simulink model "smm_gait_control"  (R2018b)
settings: configuration reference "Configuration1khz" (kept outside this file)
InitFcn:
  | addpath('./functions/')
  | addpath('./policies/')
  | control_params
values from neighbouring files (symbols this model uses):
  rest = extract_policy_variables('policies/rest.mat')    [control_params.m]
  run_slow = extract_policy_variables('policies/06_run_reduced.mat')    [control_params.m]
  walk_slow = extract_policy_variables('policies/06_walk.mat')    [control_params.m]
undefined symbols (not defined in the file or in its folder): ctrl, Discrete, initial_dx_estimate, initial_dy_estimate, initial_dz_estimate, initial_z_estimate, sample_time, Time
libraries: simulink x42, ctrlSharedLib x7
(part 5 of 5)

== matlab function smm_gait_control/Behavior/Filtering/Kalman Filtering/Measurement Noise Covariance Matricies ==
  data: R_no_position output; R_transverse_right output; R_transverse_left output; vertical_GRF_L input; vertical_GRF_R input; sample_time parameter; ctrl parameter; R_vertical output
function [R_no_position, R_transverse_right, R_transverse_left, R_vertical] =...
         MeasurementNoiseCovariance(vertical_GRF_L, vertical_GRF_R, ...
         sample_time, ctrl)

    % filter states: [dx_w]; [dy_w]; [dz_w];
    % measurements:  [dx_w-dfL + dfL_hat; dx_w-dfR + dfR_hat]; 

    ratio_L = max(0, min(vertical_GRF_L/(ctrl.kalman_stance_slip_threshold*ctrl.m_total*ctrl.g),1)); % ratio is 0 if no load, 1 if at least equilibrium
    ratio_R = max(0, min(vertical_GRF_R/(ctrl.kalman_stance_slip_threshold*ctrl.m_total*ctrl.g),1));
    R_transverse_right = diag([ratio_R*ctrl.R_kalman_foot_stance + (1-ratio_R)*ctrl.R_kalman_foot_slip, ...
                               ctrl.R_kalman_accelerometer])/sample_time;
    R_transverse_left = diag([ratio_L*ctrl.R_kalman_foot_stance + (1-ratio_L)*ctrl.R_kalman_foot_slip, ...
                              ctrl.R_kalman_accelerometer])/sample_time;            
    R_vertical = diag([ratio_L*ctrl.R_kalman_foot_stance  + (1-ratio_L)*ctrl.R_kalman_foot_slip,...
                       ratio_R*ctrl.R_kalman_foot_stance  + (1-ratio_R)*ctrl.R_kalman_foot_slip,...
                       ctrl.R_kalman_accelerometer])/sample_time;
                   
    R_no_position = diag([ratio_L*ctrl.R_kalman_dfoot_stance + (1-ratio_L)*ctrl.R_kalman_dfoot_slip, ...
                          ratio_R*ctrl.R_kalman_dfoot_stance + (1-ratio_R)*ctrl.R_kalman_dfoot_slip, ...
                          ctrl.R_kalman_accelerometer])/sample_time;
end

== matlab function smm_gait_control/Behavior/Convert to Body Frame IMU Accelerations ==
  data: accelerometer input; imu_accelerations output; ctrl parameter
function imu_accelerations = imu_to_body_frame(accelerometer, ctrl)
    z_up_rotation = [1, 0, 0; 0, 0, 1; 0, -1, 0];
    align_xy_rotation = [sqrt(2)/2, -sqrt(2)/2, 0; sqrt(2)/2, sqrt(2)/2, 0; 0, 0, 1];
    imu_accelerations = ctrl.g*z_up_rotation*align_xy_rotation*accelerometer;
end

== matlab function smm_gait_control/Behavior/Motion Planner/Plan Swing Leg Trajectories/Plan Swing Trajectories ==
  data: enable input; replan input; angle_of_attack input; touchdown_will_occur input; plan_length input; stance_plan_timings input size=[ctrl.max_trajectory_length 1]; stance_state_plan input size=[ctrl.max_trajectory_length 6]; double_support_time input; t_plan input; section_number input; phase input; com_x_velocity input; z_state input; foot2com_x_primary input; foot2com_z_primary input; foot2com_x_secondary input; foot2com_z_secondary input; right_is_primary input; gait_id input; neutral_point input; k_placement input; desired_x_primary output; desired_y_primary output; desired_z_primary output; desired_x_secondary output; desired_y_secondary output; desired_z_secondary output; ctrl parameter; walk_slow parameter; run_slow parameter; rest parameter
% Plan Foot2CoM trajectories in XYZ space for the swing phase
function [desired_x_primary, desired_y_primary, desired_z_primary, ...
          desired_x_secondary, desired_y_secondary, desired_z_secondary] = ...
          PlanFeet(enable, replan, angle_of_attack, touchdown_will_occur, ...
                    plan_length, stance_plan_timings, stance_state_plan, double_support_time, t_plan, ...
                    section_number, phase, com_x_velocity, z_state, ...
                    foot2com_x_primary, foot2com_z_primary, ...
                    foot2com_x_secondary, foot2com_z_secondary, ...
                    right_is_primary, gait_id, neutral_point, k_placement, ...
                    ctrl, walk_slow, run_slow, rest)
                  
  % not applicable in double support (return zero)
  if phase == 2
    desired_x_primary = [0 0 0]';
    desired_y_primary = [0 0 0]';
    desired_z_primary = [0 0 0]';
    desired_x_secondary = [0 0 0]';
    desired_y_secondary = [0 0 0]';
    desired_z_secondary = [0 0 0]';
    return;
  end
  
  % select gait dependent parameters
  switch(gait_id)
    case 1
      com_x_vel_desired = rest.desired_x_velocity;
      rest_length = rest.model.l0;
    case 2
      com_x_vel_desired = walk_slow.desired_x_velocity;
      rest_length = walk_slow.model.l0;
    case 3
      com_x_vel_desired = run_slow.desired_x_velocity;
      rest_length = run_slow.model.l0;
    otherwise
      com_x_vel_desired = run_slow.desired_x_velocity;
      rest_length = run_slow.model.l0;
  end
  
  % persistent variables to store swing foot plan(s) as splines in (X,Z) space
  persistent ax1 bx1 cx1 dx1 ax2 bx2 cx2 dx2 az1 bz1 cz1 dz1 az2 bz2 cz2 dz2 ...
             t_final x0_secondary_pos x0_secondary_vel

  % plan swing feet
  if isempty(ax1) || replan
    % convert (leg_length, leg_angle) space to (X,Z) space
    x_target = -rest_length * cosd(angle_of_attack);
    z_target =  rest_length * sind(angle_of_attack);
    if section_number == 1 % Flight (plan primary and secondary legs)
      % calculate swing time in flight
      t_final = (z_state(2) + sqrt(max(z_state(2)^2 - 2*ctrl.g*(z_target-z_state(1)),0)))/ctrl.g;
      t_min = abs(z_target - foot2com_z_primary(1)) / ctrl.max_vert_swing_speed;
      t_final = max(t_final, t_min); % lower bound swing time
      % primary x trajectory during flight
      x0_primary_pos = foot2com_x_primary(1); 
      x0_primary_vel = foot2com_x_primary(2);
      xf_pos = x_target;
      xf_vel = com_x_velocity; % match horizontal ground speed in flight
      [ ax1, bx1, cx1, dx1 ] = FindCubicCoefficients( x0_primary_pos, x0_primary_vel, ...
                                                      xf_pos, xf_vel, t_final );
      % secondary x trajectory during flight (symmetric about x = 0)
      x0_secondary_pos = foot2com_x_secondary(1); 
      x0_secondary_vel = foot2com_x_secondary(2);
      xf_pos = -x_target;
      xf_vel = 0;
      [ ax2, bx2, cx2, dx2 ] = FindCubicCoefficients( x0_secondary_pos, x0_secondary_vel, ...
                                                      xf_pos, xf_vel, t_final );
      % primary z trajectory during flight
      z0_pos = foot2com_z_primary(1);
      z0_vel = foot2com_z_primary(2);
      zf_pos = z_target;
      zf_vel = 0;
      [ az1, bz1, cz1, dz1 ] = FindCubicCoefficients( z0_pos, z0_vel, zf_pos, zf_vel, t_final );
      % secondary z trajectory during flight
      z0_pos = foot2com_z_secondary(1);
      z0_vel = foot2com_z_secondary(2);
      zf_pos = z_target - ctrl.z_retract_flight;
      zf_vel = 0;
      [ az2, bz2, cz2, dz2 ] = FindCubicCoefficients( z0_pos, z0_vel, zf_pos, zf_vel, t_final );
    elseif section_number == 2 % single support initial (SSI)
      final_stance_time = stance_plan_timings(plan_length);
      % plan targets based on if transitioning to double support or flight
      if touchdown_will_occur % to double support phase
        t_final = max(double_support_time, ctrl.min_swing_time);
        zmid_retract = 0.5 * ctrl.retract_extend_speed * t_final; % approximation
        zmid_retract = max(min(zmid_retract, ctrl.max_z_retract), ctrl.min_z_retract);
        zf_pos = z_target;
      else                    % to flight phase
        t_final = final_stance_time; 
        zmid_retract = ctrl.z_retract_flight;
        zf_pos = stance_state_plan(plan_length,3) - 0.30*zmid_retract;
      end
      % secondary x trajectory
      x0_secondary_pos = foot2com_x_secondary(1); 
      x0_secondary_vel = foot2com_x_secondary(2);
      xf_pos = x_target;
      xf_vel = 0;
      [ ax1, bx1, cx1, dx1 ] = FindCubicCoefficients( x0_secondary_pos, x0_secondary_vel, ...
                                                      xf_pos, xf_vel, t_final );
      ax2 = 0; bx2 = 0; cx2 = 0; dx2 = 0;
      % (retract/extend from SSI) 
      % secondary z trajectory (first half, retraction)
      z0_pos = foot2com_z_secondary(1);
      z0_vel = foot2com_z_secondary(2);
      zmid_pos = interp1(stance_plan_timings(1:plan_length), stance_state_plan(1:plan_length,3), ...
                         min(0.5*t_final, final_stance_time),'linear') - zmid_retract;
      zmid_vel = 0;
      [ az1, bz1, cz1, dz1 ] = FindCubicCoefficients( z0_pos, z0_vel, zmid_pos, zmid_vel, 0.5*t_final );
      % secondary z trajectory (second half, extension)
      zf_vel = 0;
      [ az2, bz2, cz2, dz2 ] = FindCubicCoefficients( zmid_pos, zmid_vel, zf_pos, zf_vel, 0.5*t_final );
    else % section_number == 3, single support apex (SSA)
      % plan until initial double support
      min_time = abs(z_target - foot2com_z_secondary(1)) / ctrl.retract_extend_speed;
      t_final = max(double_support_time, min_time);
      % secondary x trajectory
      x0_secondary_pos = foot2com_x_secondary(1); 
      x0_secondary_vel = foot2com_x_secondary(2);
      xf_pos = x_target;
      xf_vel = 0;
      [ ax1, bx1, cx1, dx1 ] = FindCubicCoefficients( x0_secondary_pos, x0_secondary_vel, ...
                                                      xf_pos, xf_vel, t_final );
      ax2 = 0; bx2 = 0; cx2 = 0; dx2 = 0;
      % secondary z trajectory (only extend from SSA)
      z0_pos = foot2com_z_secondary(1);
      z0_vel = foot2com_z_secondary(2);
      zf_vel = 0;
      [ az1, bz1, cz1, dz1 ] = FindCubicCoefficients( z0_pos, z0_vel, z_target, zf_vel, t_final );
      az2 = 0; bz2 = 0; cz2 = 0; dz2 = 0;
    end
  end
  
  % y target varies from left to right side of robot
  if right_is_primary
    y_swing_target_1 = ctrl.y_swing_target_right;
    y_swing_target_2 = ctrl.y_swing_target_left;
  else
    y_swing_target_1 = ctrl.y_swing_target_left;
    y_swing_target_2 = ctrl.y_swing_target_right;
  end
  
  % compute reference from polynomials if enabled
  if enable
    % bound the time
    trajectory_valid = t_plan <= t_final;
    t_plan = min(max(t_plan,0),t_final);
%     % replan using feedback policy
%     if phase == 1 && touchdown_will_occur
%        %xf_pos = neutral_point + k_placement * (com_x_vel_desired - com_x_velocity);
%        xf_pos = -0.25 + 0.10 * (com_x_vel_desired - com_x_velocity);
%        xf_pos = min(max(xf_pos, -0.5), 0.5);
%        xf_vel = 0;
%       [ ax1, bx1, cx1, dx1 ] = FindCubicCoefficients( x0_secondary_pos, x0_secondary_vel, xf_pos, xf_vel, t_final );
%     end
    % compute x reference
    x_pos = ax1*t_plan^3 + bx1*t_plan^2 + cx1*t_plan + dx1;
    x_vel = trajectory_valid*(3*ax1*t_plan^2 + 2*bx1*t_plan + cx1);
    x_acc = trajectory_valid*(6*ax1*t_plan + 2*bx1);
    % compute other references in flight
    if phase == 0
        x_pos_2 = ax2*t_plan^3 + bx2*t_plan^2 + cx2*t_plan + dx2;
        x_vel_2 = trajectory_valid*(3*ax2*t_plan^2 + 2*bx2*t_plan + cx2);
        x_acc_2 = trajectory_valid*(6*ax2*t_plan + 2*bx2);
        z_pos_1 = az1*t_plan^3 + bz1*t_plan^2 + cz1*t_plan + dz1;
        z_vel_1 = trajectory_valid*(3*az1*t_plan^2 + 2*bz1*t_plan + cz1);
        z_acc_1 = trajectory_valid*(6*az1*t_plan + 2*bz1);
        z_pos_2 = az2*t_plan^3 + bz2*t_plan^2 + cz2*t_plan + dz2;
        z_vel_2 = trajectory_valid*(3*az2*t_plan^2 + 2*bz2*t_plan + cz2);
        z_acc_2 = trajectory_valid*(6*az2*t_plan + 2*bz2); 
        % assign references to outputs
        desired_x_primary = [x_pos; x_vel; x_acc];
        desired_y_primary = [y_swing_target_1; 0; 0];
        desired_z_primary = [z_pos_1; z_vel_1; z_acc_1];
        desired_x_secondary = [x_pos_2; x_vel_2; x_acc_2];
        desired_y_secondary = [y_swing_target_2; 0; 0];
        desired_z_secondary = [z_pos_2; z_vel_2; z_acc_2];
    else % compute z references in single support
      if section_number == 2
        if t_plan < 0.5*t_final % retraction (always retract)
          z_pos = az1*t_plan^3 + bz1*t_plan^2 + cz1*t_plan + dz1;
          z_vel = trajectory_valid*(3*az1*t_plan^2 + 2*bz1*t_plan + cz1);
          z_acc = trajectory_valid*(6*az1*t_plan + 2*bz1); 
        else % extension
          t_plan = t_plan - 0.5*t_final;
          z_pos = az2*t_plan^3 + bz2*t_plan^2 + cz2*t_plan + dz2;
          z_vel = trajectory_valid*(3*az2*t_plan^2 + 2*bz2*t_plan + cz2);
          z_acc = trajectory_valid*(6*az2*t_plan + 2*bz2);
        end
      else % section_number == 3
        z_pos = az1*t_plan^3 + bz1*t_plan^2 + cz1*t_plan + dz1;
        z_vel = trajectory_valid*(3*az1*t_plan^2 + 2*bz1*t_plan + cz1);
        z_acc = trajectory_valid*(6*az1*t_plan + 2*bz1); 
      end
      if touchdown_will_occur && ~trajectory_valid
        z_pos = z_pos + 0.05;
      end
      % assign references to outputs
      desired_x_primary = [0; 0; 0];
      desired_y_primary = [0; 0; 0];
      desired_z_primary = [0; 0; 0];
      desired_x_secondary = [x_pos; x_vel; x_acc];
      desired_y_secondary = [y_swing_target_2; 0; 0];
      desired_z_secondary = [z_pos; z_vel; z_acc];
    end

  else % Use static targets otherwise
    desired_y_primary = [y_swing_target_1 0 0]';
    desired_y_secondary = [y_swing_target_2 0 0]';
    
    % single support static target
    desired_x_primary = [ctrl.static_single_x_pos_swing 0 0]';
    desired_z_primary = [ctrl.static_single_z_pos_swing 0 0]';
    desired_x_secondary = -desired_x_primary;
    desired_z_secondary = desired_z_primary - ctrl.z_retract_flight;
    
    % double support static target
    if gait_id == 1
      desired_z_primary = [ctrl.static_double_z_pos_swing 0 0]';
      desired_z_secondary = desired_z_primary;
      if phase == 1 % single support
        desired_x_primary = [0; 0; 0];
        desired_x_secondary = [-sign(foot2com_x_primary(1)) * abs(ctrl.static_double_x_pos_swing); 0; 0];
      else          % flight
        desired_x_primary = [ctrl.static_double_x_pos_swing 0 0]';
        desired_x_secondary = -desired_x_primary;
      end
    end
    
  end
  
end

== matlab function smm_gait_control/Behavior/SEA Measurements/Leg Dynamics Left ==
  data: tau_back input; tau_front input; axial_force output; leg_width input; leg_length input; ortho_force output
function [axial_force, ortho_force] = fcn(tau_back, tau_front, leg_width, leg_length)

  % prevent divide by zero
  leg_width(1) = max(leg_width(1),eps);
  leg_length(1) = max(leg_length(1),eps);

  % forces and torques
  hip_torque = tau_front + tau_back;
  spread_torque = tau_front - tau_back;
  axial_force = zeros(2,1);
  axial_force(1) = spread_torque(1) / leg_width(1);
  ortho_force = zeros(2,1);
  ortho_force(1) = hip_torque(1) / leg_length(1);
  
  % time derivatives
  axial_force(2) = (leg_width(1)*spread_torque(2) - spread_torque(1)*leg_width(2)) / (leg_width(1)*leg_width(1));
  ortho_force(2) = (leg_length(1)*hip_torque(2) - hip_torque(1)*leg_length(2)) / (leg_length(1)*leg_length(1));
  
end

== matlab function smm_gait_control/Behavior/Leg Plane GRF Right/World Frame React Forces ==
  data: F_horz output; leg_angle input; F_vert output; torso_pitch input; F_axial input; F_ortho input
function [F_horz, F_vert] = fcn(leg_angle, torso_pitch, F_axial, F_ortho)

  % define world frame leg angle
  gamma = leg_angle + torso_pitch;

  % compute forces
  F_vert = zeros(2,1);
  F_horz = zeros(2,1);
  F_vert(1) = -F_axial(1)*cos(gamma(1)) + F_ortho(1)*sin(gamma(1));
  F_horz(1) = -F_axial(1)*sin(gamma(1)) - F_ortho(1)*cos(gamma(1));
  
  % compute time derivatives
  F_vert(2) =  gamma(2)*(F_axial(1)*sin(gamma(1)) + F_ortho(1)*cos(gamma(1))) - F_axial(2)*cos(gamma(1)) + F_ortho(2)*sin(gamma(1));
  F_horz(2) =  gamma(2)*(-F_axial(1)*cos(gamma(1)) + F_ortho(1)*sin(gamma(1))) - F_axial(2)*sin(gamma(1)) - F_ortho(2)*cos(gamma(1));
  
end

== matlab function smm_gait_control/Behavior/Leg Plane GRF Left/World Frame React Forces ==
  data: F_horz output; leg_angle input; F_vert output; torso_pitch input; F_axial input; F_ortho input
function [F_horz, F_vert] = fcn(leg_angle, torso_pitch, F_axial, F_ortho)

  % define world frame leg angle
  gamma = leg_angle + torso_pitch;

  % compute forces
  F_vert = zeros(2,1);
  F_horz = zeros(2,1);
  F_vert(1) = -F_axial(1)*cos(gamma(1)) + F_ortho(1)*sin(gamma(1));
  F_horz(1) = -F_axial(1)*sin(gamma(1)) - F_ortho(1)*cos(gamma(1));
  
  % compute time derivatives
  F_vert(2) =  gamma(2)*(F_axial(1)*sin(gamma(1)) + F_ortho(1)*cos(gamma(1))) - F_axial(2)*cos(gamma(1)) + F_ortho(2)*sin(gamma(1));
  F_horz(2) =  gamma(2)*(-F_axial(1)*cos(gamma(1)) + F_ortho(1)*sin(gamma(1))) - F_axial(2)*sin(gamma(1)) - F_ortho(2)*cos(gamma(1));
  
end

== matlab function smm_gait_control/Behavior/Swing Leg Control Secondary/Virtual Leg to Four Bar ==
  data: l_leg input; dl_leg input; ddl_leg input; phi input; dphi input; ddphi input; back output; dback output; ddback output; front output; dfront output; ddfront output
function [back, dback, ddback, front, dfront, ddfront] = VirtualLegToFourBar(l_leg, dl_leg, ddl_leg, phi, dphi, ddphi)
    [back, dback, ddback, front, dfront, ddfront] = VirtualLegToFourBar(l_leg, dl_leg, ddl_leg, phi, dphi, ddphi);
end

== matlab function smm_gait_control/Behavior/CoM Kinematics/PositionUsingRobotGeometry ==
  data: com_left_yawed output; dcom_left_yawed output; com_right_yawed output; dcom_right_yawed output; roll input; pitch input; yaw input; left_leg_sagittal_angle input; left_leg_lateral_angle input; left_leg_length input; right_leg_sagittal_angle input; right_leg_lateral_angle input; right_leg_length input; com_left_global output; dcom_left_global output; ctrl parameter; com_right_global output; dcom_right_global output; com_pelvis_body output; dcom_pelvis_body output
% Returns CoM relative to primary foot
function [com_left_yawed, dcom_left_yawed, ...
          com_right_yawed, dcom_right_yawed, ...
          com_left_global, dcom_left_global, ...
          com_right_global, dcom_right_global, ...
          com_pelvis_body, dcom_pelvis_body] = ...
         ComPositionUsingRobotGeometry(roll, pitch, yaw, ...
                           left_leg_sagittal_angle, left_leg_lateral_angle, left_leg_length, ...
                           right_leg_sagittal_angle, right_leg_lateral_angle, right_leg_length, ...
                           ctrl)
                    
  q =  [roll(1), pitch(1), yaw(1), ...
        left_leg_sagittal_angle(1), left_leg_lateral_angle(1), left_leg_length(1), ...
        right_leg_sagittal_angle(1), right_leg_lateral_angle(1), right_leg_length(1)];
  dq = [roll(2), pitch(2), yaw(2), ...
        left_leg_sagittal_angle(2), left_leg_lateral_angle(2), left_leg_length(2), ...
        right_leg_sagittal_angle(2), right_leg_lateral_angle(2), right_leg_length(2)];

  [ com_pelvis, dcom_pelvis, ...
    com_left, dcom_left, ...
    com_right, dcom_right ] = ...
  ComCalculationFromRobot( q, dq, ctrl.m_torso, ctrl.m_leg_motor, ctrl.m_leg, ctrl.com_torso, ...
                           ctrl.com_leg_motor, ctrl.lateral_offset );
  
  % left foot measurements
  com_left_yawed = com_left(4:6);
  com_left_global = com_left(7:9);
  dcom_left_yawed = dcom_left(4:6);
  dcom_left_global = dcom_left(7:9);
  
  % right foot measurements
  com_right_yawed = com_right(4:6);
  com_right_global = com_right(7:9);
  dcom_right_yawed = dcom_right(4:6);
  dcom_right_global = dcom_right(7:9);
  
  % pelvis measurement
  com_pelvis_body = com_pelvis(1:3);
  dcom_pelvis_body = dcom_pelvis(1:3);
  
end

== matlab function smm_gait_control/Behavior/Primary-Secondary Routing Outputs ==
  data: right_is_primary input size=1; joint_torque_primary input size=2; motor_velocity_primary input size=2; lateral_torque_primary input size=1; joint_torque_secondary input size=2; motor_velocity_secondary input size=2; lateral_torque_secondary input size=1; joint_torque_right output size=2; motor_velocity_right output size=2; lateral_torque_right output size=1; joint_torque_left output size=2; motor_velocity_left output size=2; lateral_torque_left output size=1
% Switch between "primary" and "secondary" leg variables
function [joint_torque_right, ...
          motor_velocity_right, ...
          lateral_torque_right, ...
          joint_torque_left, ...
          motor_velocity_left, ...
          lateral_torque_left] ...
          = SignalSwitch(...
          right_is_primary, ...
          joint_torque_primary, ...
          motor_velocity_primary, ...
          lateral_torque_primary, ...
          joint_torque_secondary, ...
          motor_velocity_secondary, ...
          lateral_torque_secondary)

if right_is_primary % right leg is primary
  joint_torque_right = joint_torque_primary;
  motor_velocity_right = motor_velocity_primary;
  lateral_torque_right = lateral_torque_primary;
  joint_torque_left = joint_torque_secondary;
  motor_velocity_left = motor_velocity_secondary;
  lateral_torque_left = lateral_torque_secondary;
else % left leg is primary
  joint_torque_right = joint_torque_secondary;
  motor_velocity_right = motor_velocity_secondary;
  lateral_torque_right = lateral_torque_secondary;
  joint_torque_left = joint_torque_primary;
  motor_velocity_left = motor_velocity_primary;
  lateral_torque_left = lateral_torque_primary;
end

== matlab function smm_gait_control/Behavior/Swing Leg Control Primary/Avoid Hitting Mechanical Limits ==
  data: back_cmd output double; front_cmd output double; dback_cmd output double; dfront_cmd output double; ddback_cmd output double; ddfront_cmd output double; back_desired input; dback_desired input; ddback_desired input; front_desired input; dfront_desired input; ddfront_desired input; ctrl parameter
%% Avoid fourbar limits by saturating the commands and ensuring we don't command velocities or 
% accelerations that would push us into the limits when nearby
function [back_cmd, front_cmd, dback_cmd, dfront_cmd, ddback_cmd, ddfront_cmd] ...
    = AvoidFourbarLimits(back_desired,dback_desired, ddback_desired, ...
          front_desired, dfront_desired, ddfront_desired, ...
          ctrl)
    [back_cmd, front_cmd, dback_cmd, dfront_cmd, ddback_cmd, ddfront_cmd] = ...
      AvoidFourbarLimits(back_desired, dback_desired, ddback_desired, ...
                         front_desired, dfront_desired, ddfront_desired, ...
                         ctrl.min_front_bar_angle, ctrl.max_front_bar_angle, ...
                         ctrl.min_back_bar_angle, ctrl.max_back_bar_angle);
end

== matlab function smm_gait_control/Behavior/Swing Leg Control Secondary/Avoid Virtual Leg Length Limits ==
  data: l_leg_desired input; dl_leg_desired input; ddl_leg_desired input; l_leg_cmd output double; dl_leg_cmd output double; ddl_leg_cmd output double; ctrl parameter
%% Avoid virtual leg length limits by ensuring we don't command position/velocities/accelerations that would hit them.
function [l_leg_cmd, dl_leg_cmd, ddl_leg_cmd] = ...
  AvoidVirtualLengthLimits(l_leg_desired, dl_leg_desired, ddl_leg_desired, ctrl)
    [l_leg_cmd, dl_leg_cmd, ddl_leg_cmd] = ...
      AvoidVirtualLengthLimits(l_leg_desired, dl_leg_desired, ddl_leg_desired, ...
                               ctrl.min_leg_length, ctrl.max_leg_length);
end

== matlab function smm_gait_control/Behavior/Swing Leg Control Primary/Avoid Virtual Leg Length Limits ==
  data: l_leg_desired input; dl_leg_desired input; ddl_leg_desired input; l_leg_cmd output double; dl_leg_cmd output double; ddl_leg_cmd output double; ctrl parameter
%% Avoid virtual leg length limits by ensuring we don't command position/velocities/accelerations that would hit them.
function [l_leg_cmd, dl_leg_cmd, ddl_leg_cmd] = ...
  AvoidVirtualLengthLimits(l_leg_desired, dl_leg_desired, ddl_leg_desired, ctrl)
    [l_leg_cmd, dl_leg_cmd, ddl_leg_cmd] = ...
      AvoidVirtualLengthLimits(l_leg_desired, dl_leg_desired, ddl_leg_desired, ...
                               ctrl.min_leg_length, ctrl.max_leg_length);
end

== matlab function smm_gait_control/Behavior/Swing Leg Control Primary/Convert CoM (X,Y,Z) to  (Leg Angles, Leg Length) ==
  data: desired_leg_length output; X_star input; Y_star input; Z_star input; right_left input; pelvis2com_pos input; desired_alpha output; desired_beta output; pelvis2com_vel input; roll input; pitch input; sagittal_angle input; lateral_angle input; leg_length input; ctrl parameter
%% Convert Foot2CoM vector from (X, Y, Z) to (leg length, leg angle) space
function [ desired_leg_length, desired_alpha, desired_beta ]  =  ...
          ConvertToJointAnglesAndLegLength(X_star, Y_star, Z_star, right_left,...
                           pelvis2com_pos, pelvis2com_vel, ...
                           roll, pitch, sagittal_angle, lateral_angle, leg_length,...
                           ctrl) 

    q = [roll(1), pitch(1), sagittal_angle(1), lateral_angle(1), leg_length(1)];
    dq = [roll(2), pitch(2), sagittal_angle(2), lateral_angle(2), leg_length(2)];
    [desired_alpha, desired_beta, desired_leg_length] = ...
      ConvertComPositionToLegAnglesAndLegLength(X_star, Y_star, Z_star, right_left, ...
                                                pelvis2com_pos, pelvis2com_vel, ...
                                                q, dq, ctrl.lateral_offset);
    desired_beta = saturate(desired_beta, ctrl.min_lateral_beta, ctrl.max_lateral_beta);
end

function [desired_saturated] = saturate(desired, min_lateral_beta, max_lateral_beta)
    desired_saturated = desired;
    if desired(1) < min_lateral_beta
        desired_saturated = [min_lateral_beta; 0; 0];
    elseif desired(1) > max_lateral_beta
        desired_saturated = [max_lateral_beta; 0; 0];    
    end
end

== matlab function smm_gait_control/Behavior/Swing Leg Control Primary/Virtual Leg to Four Bar ==
  data: l_leg input; dl_leg input; ddl_leg input; phi input; dphi input; ddphi input; back output; dback output; ddback output; front output; dfront output; ddfront output
function [back, dback, ddback, front, dfront, ddfront] = VirtualLegToFourBar(l_leg, dl_leg, ddl_leg, phi, dphi, ddphi)
    [back, dback, ddback, front, dfront, ddfront] = VirtualLegToFourBar(l_leg, dl_leg, ddl_leg, phi, dphi, ddphi);
end

== matlab function smm_gait_control/Behavior/Planar Inverse Dynamics/2D Inverse Dynamics ==
  data: phase input; Fx1 input; Fz1 input; Fx2 input; Fz2 input; tau_back_1 output; torso_pitch input; x_velocity input; z_velocity input; leg_angle_1 input; leg_length_1 input; leg_width_1 input; tau_rotor_f_1 input; tau_rotor_b_1 input; leg_angle_2 input; leg_length_2 input; leg_width_2 input; tau_rotor_f_2 input; tau_rotor_b_2 input; d_pelvis_to_com input; ctrl parameter; tau_front_1 output; tau_back_2 output; tau_front_2 output
%% Planar Inverse dynamics for single or double support
% Realize desired ground reaction forces using joint torques
function [tau_back_1, tau_front_1, tau_back_2, tau_front_2] = ...
            inverse_dynamics(phase, Fx1, Fz1, Fx2, Fz2, ...
                            torso_pitch, x_velocity, z_velocity, ...
                            leg_angle_1, leg_length_1, leg_width_1, ...
                            tau_rotor_f_1, tau_rotor_b_1, ...
                            leg_angle_2, leg_length_2, leg_width_2, ...
                            tau_rotor_f_2, tau_rotor_b_2, ...
                            d_pelvis_to_com, ...
                            ctrl) 
    % System variables
    g      = ctrl.g;
    N      = -ctrl.leg_mtr_gear_ratio;
    m      = ctrl.m_total;      % mass of system + boom
    m_leg  = ctrl.m_leg;
    Il     = ctrl.i_leg;        % inertia of leg
    It     = ctrl.i_robot;      % inertia of system
    d      = d_pelvis_to_com;   % distance from pelvis to system CoM
    th     = torso_pitch(1);
    dth    = torso_pitch(2);
    dx     = x_velocity;
    dz     = z_velocity;
    % Leg 1 variables
    l1     = leg_length_1(1);
    dl1    = leg_length_1(2);
    g1     = leg_angle_1(1)+torso_pitch(1);   % global leg angle
    dg1    = leg_angle_1(2)+torso_pitch(2);
    w1     = leg_width_1(1);
    t_rf1  = tau_rotor_f_1;       % torque applied at front rotor 
    t_rb1  = tau_rotor_b_1;       % torque applied at back rotor
    % Leg 2 variables
    l2     = leg_length_2(1);
    dl2    = leg_length_2(2);
    g2     = leg_angle_2(1)+torso_pitch(1);   % global leg angle
    dg2    = leg_angle_2(2)+torso_pitch(2);
    w2     = leg_width_2(1);     
    t_rf2  = tau_rotor_f_2;       % torque applied at front rotor 
    t_rb2  = tau_rotor_b_2;       % torque applied at back rotor

  % Dynamics matrices
  J  = [1  0  -d*cos(th)    sin(g1)     l1*cos(g1)     0           0;
        0  1   d*sin(th)    cos(g1)    -l1*sin(g1)     0           0;
        1  0  -d*cos(th)    0           0              sin(g2)     l2*cos(g2);
        0  1   d*sin(th)    0           0              cos(g2)    -l2*sin(g2)];

  dJ = [0  0  d*dth*sin(th)    dg1*cos(g1)    (-l1*dg1*sin(g1)+dl1*cos(g1))    0           0;
        0  0  d*dth*cos(th)   -dg1*sin(g1)    (-l1*dg1*cos(g1)-dl1*sin(g1))    0           0;
        0  0  d*dth*sin(th)    0              0                                dg2*cos(g2)    (-l2*dg2*sin(g2)+dl2*cos(g2));
        0  0  d*dth*cos(th)    0              0                               -dg2*sin(g2)    (-l2*dg2*cos(g2)-dl2*sin(g2))];

  dq  = [ dx dz dth dl1 dg1 dl2 dg2 ]';

  M = [m  0   0   0    0      0    0; 
       0  m   0   0    0      0    0;
       0  0   It  0    0      0    0;   
       0  0   0   Il   0      0    0;  
       0  0   0   0    m_leg  0    0;
       0  0   0   0    0      Il   0;
       0  0   0   0    0      0    m_leg];  

  h = [0; -m*g; (-t_rf1-t_rb1-t_rf2-t_rb2); 0; 0; 0; 0];

  S = [ 0         0          0         0;
        0         0          0         0;
        -(N-1)/N   -(N-1)/N    -(N-1)/N   -(N-1)/N;
        1/w1      -1/w1      0         0;
        1         1          0         0;
        0         0          1/w2      -1/w2;
        0         0          1         1];

  F = [Fx1, Fz1, Fx2, Fz2]';

  P = [M     -S;       
       J      zeros(4,4)];

  z = P\([h; -dJ*dq] + [J zeros(4,4)]'*F);
  
  % Extract joint torques
  tau_front_1 = z(8);
  tau_back_1 = z(9);
  tau_front_2 = z(10);
  tau_back_2 = z(11);
  
end

== matlab function smm_gait_control/Behavior/Motion Planner/Lookup Stance Control Terms ==
  data: horizon_enabled input; t_plan input; plan_length input; reference output size=[6 1]; feedback_matrix output size=[3 6]; feedforward_terms output size=[3 1]; timings input size=[ctrl.max_trajectory_length 1]; state_plan input size=[ctrl.max_trajectory_length 6]; K_lqr_plan input size=[ctrl.max_trajectory_length 3 6]; feedforward_plan input size=[ctrl.max_trajectory_length 3]; phase input; plan_phase input
%% Lookup plan terms for stance control at current time
function [ reference, feedback_matrix, feedforward_terms ] = ...
           stance_control_terms(horizon_enabled, t_plan, ...
                                plan_length, timings, state_plan, K_lqr_plan, feedforward_plan, ...
                                phase, plan_phase)
                              
  % Specify variable sizes for Simulink coder
  coder.varsize('feedback_matrix',[3,6]);
  coder.varsize('feedforward_terms',[3,1]);
  
  % Compute reference, feedback matrix, and feedforward terms when in stance                          
  if phase == 0 || phase ~= plan_phase % In flight, or plan not yet generated
    reference = zeros(6,1);
    if phase == 1
      control_width = 2;
    else
      control_width = 3;
    end
    feedback_matrix = zeros(control_width,6);
    feedforward_terms = zeros(control_width,1);
  else
    % If finite horizon LQR is enabled, find current plan output
    if horizon_enabled
      % Interp will fail is only 1 data point, special case
      if plan_length == 1
        reference = state_plan(1,:)';
        feedback_matrix = squeeze(K_lqr_plan(1,:,:));
        feedforward_terms = feedforward_plan(1,:)';
      else % Normal interpolation
        initial_plan_time = timings(1);
        final_plan_time = timings(plan_length);
        t_plan_bounded = min(max(t_plan, initial_plan_time), final_plan_time); % bound timer to plan
        reference = interp1(timings(1:plan_length), state_plan(1:plan_length,:), t_plan_bounded, 'linear')';
        feedback_matrix = squeeze(interp1(timings(1:plan_length), K_lqr_plan(1:plan_length,:,:), t_plan_bounded,'linear'));
        feedforward_terms = interp1(timings(1:plan_length), feedforward_plan(1:plan_length,:), t_plan_bounded, 'linear')';
      end
      % Resize output for single support phase
      if phase == 1
        feedback_matrix = feedback_matrix(1:2,:);
        feedforward_terms = feedforward_terms(1:2);
      end
    else % Otherwise, approximate infinite horizon LQR
      reference = state_plan(plan_length,:)';
      feedback_matrix = squeeze(K_lqr_plan(1,:,:));
      feedforward_terms = feedforward_plan(plan_length,:)';
    end
  end

end

== matlab function smm_gait_control/Behavior/Tranform Sensor Measurements to CoM Acceleration Measurement/Compute CoM Translational Acceleration ==
  data: com_acceleration_yawed output; torso_com_acceleration_yawed output; pelvis_acceleration_yawed output; torso_angular_accelerations input; imu_translational_accelerations_body input; torso_roll input; torso_pitch input; hip_roll_accelerations input; right_hip_roll input; left_hip_roll input; ctrl parameter; right_hip_acceleration_yawed output; left_hip_acceleration_yawed output
%% Compute translational acceleration of the CoM from torso accelerometer and joint encoders
% (IMU uses non-rotating measurement frame)
function [com_acceleration_yawed, torso_com_acceleration_yawed, pelvis_acceleration_yawed, ...
          right_hip_acceleration_yawed, left_hip_acceleration_yawed] ...
          = compute_com_acceleration( torso_angular_accelerations, ...
                                      imu_translational_accelerations_body, ...
                                      torso_roll, torso_pitch, ...
                                      hip_roll_accelerations, right_hip_roll, left_hip_roll, ...
                                      ctrl)
    
    % Body frame to Yawed frame rotation matrices
    R_body_to_yawed = R_pitch(torso_pitch(1))*R_roll(torso_roll(1));
    dR_body_to_yawed = dR_pitch(torso_pitch(1),torso_pitch(2))*R_roll(torso_roll(1)) + R_pitch(torso_pitch(1))*dR_roll(torso_roll(1),torso_roll(2));
    ddR_body_to_yawed = ddR_pitch(torso_pitch(1),torso_pitch(2),torso_angular_accelerations(2))*R_roll(torso_roll(1)) ...
                        + R_pitch(torso_pitch(1))*ddR_roll(torso_roll(1),torso_roll(2),torso_angular_accelerations(1)) ... 
                        + 2*dR_pitch(torso_pitch(1),torso_pitch(2))*dR_roll(torso_roll(1),torso_roll(2));
    % Compute translational acceleration of torso COM in yawed frame
    imu_to_torso_com_acceleration_yawed = ddR_body_to_yawed*(ctrl.com_torso - ctrl.pelvis_to_imu)';
    imu_acceleration_yawed = R_body_to_yawed*imu_translational_accelerations_body;
    torso_com_acceleration_yawed = imu_acceleration_yawed + imu_to_torso_com_acceleration_yawed;
    % Compute accelerations of hip COMs
    R_right_hip_to_body =     R_roll(-pi/2+right_hip_roll(1));
    dR_right_hip_to_body =   dR_roll(-pi/2+right_hip_roll(1), right_hip_roll(2));
    ddR_right_hip_to_body = ddR_roll(-pi/2+right_hip_roll(1), right_hip_roll(2), hip_roll_accelerations(1));
    R_left_hip_to_body =     R_roll(pi/2-left_hip_roll(1));
    dR_left_hip_to_body =   dR_roll(pi/2-left_hip_roll(1), -left_hip_roll(2));
    ddR_left_hip_to_body = ddR_roll(pi/2-left_hip_roll(1), -left_hip_roll(2), -hip_roll_accelerations(2));
    imu_to_pelvis_com_acceleration_yawed = ddR_body_to_yawed*(-ctrl.pelvis_to_imu)';  
    pelvis_acceleration_yawed = imu_acceleration_yawed + imu_to_pelvis_com_acceleration_yawed;
    left_hip_acceleration_yawed = pelvis_acceleration_yawed + (ddR_body_to_yawed*R_left_hip_to_body + 2*dR_body_to_yawed*dR_left_hip_to_body + R_body_to_yawed*ddR_left_hip_to_body)*ctrl.com_leg_motor';
    right_hip_acceleration_yawed = pelvis_acceleration_yawed + (ddR_body_to_yawed*R_right_hip_to_body + 2*dR_body_to_yawed*dR_right_hip_to_body + R_body_to_yawed*ddR_right_hip_to_body)*(ctrl.com_leg_motor.*[1,-1,1])';
    % Compute total system COM acceleration
    m_hip = ctrl.m_leg+ctrl.m_leg_motor;
    m_total = 2*m_hip + ctrl.m_torso;
    com_acceleration_yawed = (ctrl.m_torso*torso_com_acceleration_yawed + m_hip*(left_hip_acceleration_yawed + right_hip_acceleration_yawed))/m_total;
    
end

function R_yp = R_pitch(theta) % map from pitched to yawed
  R_yp = [cos(theta), 0, sin(theta); ...
          0, 1, 0; ...
          -sin(theta), 0, cos(theta)];
end
function dR_yp = dR_pitch(theta,dtheta)
  dR_yp = dtheta*[-sin(theta), 0, cos(theta); ...
                  0, 0, 0; ... 
                  -cos(theta), 0, -sin(theta)];
end
function ddR_yp = ddR_pitch(theta,dtheta,ddtheta)
  ddR_yp = ddtheta*[-sin(theta), 0, cos(theta); ...
                    0, 0, 0; ... 
                    -cos(theta), 0, -sin(theta)] ...
           + dtheta^2*[-cos(theta), 0, -sin(theta); ...
                     0, 0, 0; ...
                     sin(theta), 0, -cos(theta)];
end
function R_pr = R_roll(phi) % map from rolled to pitched
  R_pr = [1, 0, 0; ...
          0, cos(phi), -sin(phi); ...
          0, sin(phi), cos(phi)]; 
end
function dR_pr = dR_roll(phi,dphi)
  dR_pr = dphi*[0, 0, 0; ...
                0, -sin(phi), -cos(phi); ...
                0, cos(phi), -sin(phi)];
end
function ddR_pr = ddR_roll(phi, dphi, ddphi)
  ddR_pr = ddphi*[0, 0, 0; ...
                  0, -sin(phi), -cos(phi); ...
                  0, cos(phi), -sin(phi)] ...
           + dphi^2*[0, 0, 0; ...
                   0, -cos(phi), sin(phi);...
                   0, -sin(phi), -cos(phi)];
end
function R_gy = R_yaw(psi) % map yawed frame to global
  R_gy = [cos(psi), -sin(psi), 0; sin(psi), cos(psi), 0; 0 0 1]; 
end
function dR_gy = dR_yaw(psi,dpsi)
  dR_gy = dpsi*[-sin(psi), -cos(psi), 0; cos(psi), -sin(psi), 0; 0 0 0];
end
function ddR_gy = ddR_yaw(psi,dpsi,ddpsi)
  ddR_gy = ddpsi*[-sin(psi), -cos(psi), 0; cos(psi), -sin(psi), 0; 0 0 0] ...
           + dpsi^2*[-cos(psi), sin(psi), 0; -sin(psi), -cos(psi), 0; 0 0 0];
end
